simulink model "ARS308_RX"  (R2018b)
settings: Solver=FixedStepAuto  StartTime=0.0  StopTime=inf  FixedStep=0.005  RelTol=1e-3
PostLoadFcn:
  | if any(exist('dsrtsu_mdlpostloadfcn', 'file') ~= 0), dsrtsu_mdlpostloadfcn('Execute', bdroot); end
libraries: rtican x18
(part 1 of 4)
settings Model: DataDictionary=ARS308_RX.sldd  DSRTSU_INTERNAL_RTI_VER=540  DSRTSU_INTERNAL_RTI_TYPE=rti1401  RTICANMMDATA=struct('GeneralSetupData',struct('modelroot','F:\src_cm4sl_1221p\src_cm4sl_1221p\src_cm4sl','generalsettings',struct('filesettings',struct('destfolder',struct('Name','RTICANMM_FILES','Check',1),'buildfolder',struct('Name','.','Check',1),'AbsDestfolder',struct('Name','F:\src_cm4sl_1221p\src_cm4sl_1221p\src_cm4sl\RTICANMM_FILES'),'AbsBuildfolder',struct('Name','F:\src_cm4sl_1221p\src_cm4sl_1221p\src_cm4sl'))),'options',struct('addpaths',1,'rmpaths',1,'addtrcexclusion',logical(1),'cannavigator',struct('checkmonitoring',0),'show_usrtrc',0,'use_usrtrc',0),'advanced',struct('options',ones(1,100)),'MPSetup',{{}},'RTI',struct('Type','RTI1401','Ver','7.12','Date','02-May-2019'),'modelname','ARS308_RX','block','ARS308_RX'))  DSRTSU_INTERNAL_RTIFPGA=130  Creator=Administrator  LastModifiedBy=石丽
settings OptimizationCC: BlockReduction=off  ConditionallyExecuteInputs=off  OptimizeBlockIOStorage=off  BufferReuse=off  GlobalBufferReuse=off  ExpressionFolding=off  PassReuseOutputArgsThreshold=0  LocalBlockOutputs=off  OptimizeBlockOrder=speed  OptimizeDataStoreBuffers=off  BusAssignmentInplaceUpdate=off
settings DebuggingCC: ParameterTunabilityLossMsg=error  BusObjectLabelMismatch=none
settings HardwareCC: ProdBitPerPointer=32  ProdBitPerSizeT=32  ProdBitPerPtrDiffT=32  ProdLargestAtomicInteger=Integer  ProdEndianess=BigEndian  ProdWordSize=32  ProdHWDeviceType=Custom Processor->Custom  TargetIntDivRoundTo=Zero  TargetEndianess=BigEndian  TargetHWDeviceType=Custom Processor->Custom
settings ModelReferenceCC: ModelReferenceNumInstancesAllowed=Single
settings SFSimCC: MATLABDynamicMemAlloc=off
settings RTWCC: SystemTargetFile=rti1401.tlc  MakeCommand=make_rti  TemplateMakefile=rti1401.tmf  Description=dSPACE DS1401 Hardware Platform  GenerateReport=on  LaunchReport=on
settings CodeAppCC: OperatorAnnotations=on
settings STFCustomTargetCC: ParMdlRefBuildCompliant=on  SystemTargetFile=rti1401.tlc
settings GRTTargetCC: TargetLangStandard=C89/C90 (ANSI)  CompOptLevelCompliant=off  ConcurrentExecutionCompliant=off  CombineOutputUpdateFcns=off  MatFileLogging=off  CPPClassGenCompliant=off  UseToolchainInfoCompliant=off

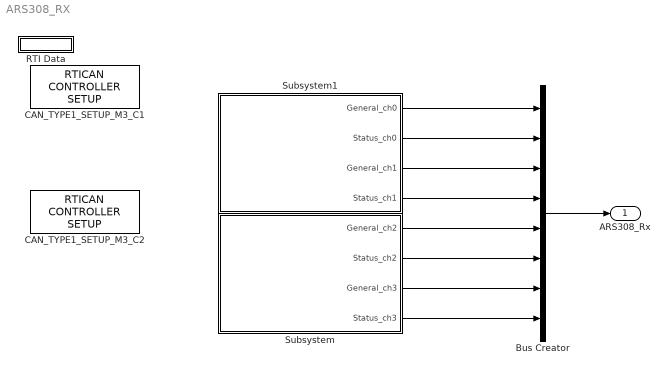
== system ARS308_RX ==
  Bus Creator : BusCreator  Inputs=8  OutDataTypeStr=Bus: ARS308_RX  NonVirtualBus=on
      settings: InheritFromInputs=off
  CAN_TYPE1_SETUP_M3_C1 : rtican/RTICAN CONTROLLER SETUP   Reserved1=[]  Reserved2=[]  Reserved3=[]  Reserved4=[]  AcceptanceMask=[]  ArbitrationField=[]  Parameters=[]  SFcnRTICANSettings=[]  MS_Struct=[]  BoardTypeNo=[]  BoardNo=[]  ChannelNo=[]  DialogFcn=[]  UnitName=[]  Revision=[]  UnitValues=[]  DSProperties=struct('RTI',struct('Version',uint32(12),'BlockType',struct('isSLSource',uint8(0),'isSLSink',uint8(0),'isHWSource',uint8(0),'isHWSink',uint8(0),'isSetup',uint8(1),'isInline',uint8(1),'isNonInline',uint8(0),'isInterrupt',uint8(0),'isChannelwise',uint8(0)),'IOBoardType','RTICAN','UnitType','NON_MESSAGE','Identifier','MASTER','DialogType','ML','BlockSet','RTICAN','SlaveProcessor','CAN'))  RTIBlockInterface=struct('InputPortsWidth',int32(0),'InputPortsActive',0,'OutputPortsWidth',int32(0),'OutputPortsActive',0,'DialogFcn','rtican_master_setup_gui','BlockDisplay',{{['CAN CONTROLLER\n SETUP'],'center'}},'IconTransparency','on','InitLevel',3,'IWork',{{{'',uint32(2)}}},'BlockName',struct('Token',{{'CAN_TYPE','_SETUP_M','_C'}},'BlockParam',{{'BoardTypeNo','BoardNo','ChannelNo'}}),'ParameterTunableNames',{{}})  RTIBlockParameters="struct('BoardTypeNo',{{1,'OFF',[]}},'BoardNo',{{3,'ON',[1 16]}},'ChannelNo',{{1,'ON',[1 2]}},'AcceptanceMask',{{0,'OFF',[]}},'ArbitrationField',{{0,'OFF',[]}},'Parameters',{{struct('Config',struct('Baudrate',500,'SampleMode',1,'UsedParamSet',1,'validSettings',1,'isBTRvalues',0,'Advanced',struct('Baudrate',{500,500,500},'Frequency',{24000000,36000000,64000000},'Settings',{struct('SMPL',0,'BRP',0,'NBT',24,'TSEG1',15,'TSEG2',6,'SJW',3,'SP',70),struct('SMPL',0,'BRP',1,'NBT',18,'TSEG1',14,'TSEG2',1,'SJW',1,'SP',88),struct('SMPL',0,'BRP',3,'NBT',16,'TSEG1',12,'TSEG2',1,'SJW',1,'SP',87)},'BTR0',{192,65,67},'BTR1',{111,30,28})),'configType',1,'Options',struct('DataFileSelected',1,'DataFileName',{{['c:\\users\\石丽\\desktop\\zone\\2020_demo\\308\\ars408_can_database_ch0 -new.dbc'],'c:\\users\\石丽\\desktop\\zone\\2020_demo\\308\\ars408_can_database_ch1-new.dbc'}},'DataFileDate',{{['18-12月-2020 14:05:27'],['18-12月-2020 14:05:27']}},'InterfaceFcn','rtican_dbc_file_parser','InterfaceFcnFileName','','LabelConfigType','volatile','AcceptanceMaskSelected',0,'MsgDataType','AllwaysDouble','NumType','hex','MaskType','STD','AcceptanceMask',0,'ArbitrationField',0,'UseMultipleMessageAccess',1),'RxReceiveStdOptions',struct('RxServiceStdEnabled',0,'RxServiceStdMsgIdent',1000,'RxServiceStdIdentNumType',1,'RxServiceStdIdentMask',0,'RxServiceStdMaskNumType',1,'RxServiceStdQueueSize',64),'RxReceiveXtdOptions',struct('RxServiceXtdEnabled',0,'RxServiceXtdMsgIdent',1001,'RxServiceXtdIdentNumType',1,'RxServiceXtdIdentMask',0,'RxServiceXtdMaskNumType',1,'RxServiceXtdQueueSize',64),'PartialNetworkingOptions',struct('switchedon',0,'format',1,'idmask',['    XXXXX XXXXXXXX XXXXXXXX XXXXXXXX'],'idcode','0','idfilter','0','datamaskused',0,'datalength',1,'datamask','0x0000000000000000','partialnetworkenable',0),'general',struct('Termination_common',1,'Termination_C252',1,'BusConfigurationRegister',0,'Transceiver','ISO11898','isFromLib',0)),'OFF',[]}},'CCPParameters',{{struct('CRO',struct('Format','STD','NumFormat','hex','Id',1639),'DTO',struct('Format','STD','NumFormat','hex','Id',2017),'StationAdr',struct('NumFormat','hex','Value',57),'StationId',struct('Value',['dSPACE CCP Service']),'Enabled',0),'OFF',[]}},'XCPParameters',{{struct('MASTER',struct('Format','STD','NumFormat','hex','Id',256),'SLAVE',struct('Format','STD','NumFormat','hex','Id',510),'Enabled',0,'PIDTransmissionEnabled',0),'OFF',[]}},'GroupId',{{struct('Group',{{'RTICAN'}},'No',2,'Behavior',{{'EVER'}},'BlockType',{{'SOURCE'}},'NameChangeFlag',1),'OFF',[]}},'SFcnRTICANSettings',{{struct('Baudrate',500,'configType',1,'AdvancedConfig',struct('Frequency',{},'BTR0',{},'BTR1',{}),'UsedParamSet',1,'STDMaskSelected','no','XTDMaskSelected','no','BoardType','DS1','BoardNo',3,'ControllerNo',1,'Transceiver','ISO11898','BusConfigRegister',0,'TerminationRes',120,'UseMultipleMessageAccess','yes','STDRXSrvcUsed','no','STDRXSrvcMsgId',1000,'STDRXSrvcMsgMask',0,'STDRXSrvcQueueSize',64,'XTDRXSrvcUsed','no','XTDRXSrvcMsgId',1001,'XTDRXSrvcQueueSize',64,'XTDRXSrvcMsgMask',0,'PN_IsPNTransciever',0,'PN_IsPNEnabled',0,'PN_MsgFormat',1,'PN_idcode',0,'PN_idmask',2047,'PN_datamaskused',0,'PN_datalength',0,'PN_datamask',['0xFF, 0xFF, 0xFF, 0xFF, 0xFF, 0xFF, 0xFF, 0xFF']),'OFF',[]}},'SFcnRTICCPSettings',{{struct('CRO',struct('Format','STD','NumFormat','hex','Id',1639),'DTO',struct('Format','STD','NumFormat','hex','Id',2017),'StationAdr',struct('NumFormat','hex','Value',57),'StationId',struct('Value',['dSPACE CCP Service']),'Enabled',0),'OFF',[]}},'SFcnRTIXCPSettings',{{struct('MASTER',struct('Format','STD','NumFormat','hex','Id',256),'SLAVE',struct('Format','STD','NumFormat','hex','Id',510),'Enabled',0,'PIDTransmissionEnabled',0),'OFF',[]}},'TLCFileName',{{'rtican_master_setup','OFF',[]}})"  RTISFcnParameters=struct('SFcnRTICANSettings','struct','SFcnRTICCPSettings','struct','SFcnRTIXCPSettings','struct','AcceptanceMask','int32','ArbitrationField','int32','TLCFileName','char')  RTIBlockParaDefault="struct('BoardTypeNo',4302,'BoardNo',1,'ChannelNo',1,'AcceptanceMask',0,'ArbitrationField',0,'Parameters',struct('Config',struct('Baudrate',500,'SampleMode',1,'UsedParamSet',1,'validSettings',1,'isBTRvalues',0,'Advanced',struct('Frequency',16000000,'BTR0',64,'BTR1',28,'Settings',struct('SMPL',0,'BRP',0,'NBT',16,'TSEG1',12,'TSEG2',1,'SJW',1,'SP',87))),'configType',1,'Options',struct('DataFileSelected',0,'DataFileName',{{['<no datafile support>']}},'DataFileDate',{{''}},'InterfaceFcn','rtican_dbc_file_parser','InterfaceFcnFileName','','LabelConfigType','volatile','AcceptanceMaskSelected',0,'MsgDataType','AllwaysDouble','NumType','hex','MaskType','STD','AcceptanceMask',0,'ArbitrationField',0,'UseMultipleMessageAccess',0),'RxReceiveStdOptions',struct('RxServiceStdEnabled',0,'RxServiceStdMsgIdent',1000,'RxServiceStdIdentNumType',1,'RxServiceStdIdentMask',0,'RxServiceStdMaskNumType',1,'RxServiceStdQueueSize',64),'RxReceiveXtdOptions',struct('RxServiceXtdEnabled',0,'RxServiceXtdMsgIdent',1001,'RxServiceXtdIdentNumType',1,'RxServiceXtdIdentMask',0,'RxServiceXtdMaskNumType',1,'RxServiceXtdQueueSize',64),'PartialNetworkingOptions',struct('switchedon',0,'format',1,'idmask',['    XXXXX XXXXXXXX XXXXXXXX XXXXXXXX'],'idcode','0','idfilter','0','datamaskused',0,'datalength',1,'datamask','0x0000000000000000','partialnetworkenable',0),'general',struct('Termination_common',1,'Termination_C252',1,'BusConfigurationRegister',0,'Transceiver','ISO11898','isFromLib',1)),'CCPParameters',struct('CRO',struct('Format','STD','NumFormat','hex','Id',1639),'DTO',struct('Format','STD','NumFormat','hex','Id',2017),'StationAdr',struct('NumFormat','hex','Value',57),'StationId',struct('Value',['dSPACE CCP Service']),'Enabled',0),'XCPParameters',struct('MASTER',struct('Format','STD','NumFormat','hex','Id',256),'SLAVE',struct('Format','STD','NumFormat','hex','Id',510),'Enabled',0,'PIDTransmissionEnabled',0),'GroupId',struct('Group',{{'RTICAN'}},'No',1,'Behavior',{{'EVER'}},'BlockType',{{'SOURCE'}},'NameChangeFlag',1),'SFcnRTICANSettings',struct('Baudrate',500,'configType',1,'AdvandedConfig',struct('Frequency',16000000,'BTR0','0x40','BTR1','0x1C'),'UsedParamSet',1,'STDMaskSelected','no','XTDMaskSelected','no','BoardType','DS4302','BoardNo',1,'ControllerNo',1,'Transceiver','ISO11898','BusConfigRegister',0,'TerminationRes',120,'UseMultipleMessageAccess','no','STDRXSrvcUsed','no','STDRXSrvcMsgId',1000,'STDRXSrvcMsgMask',0,'STDRXSrvcQueueSize',64,'XTDRXSrvcUsed','no','XTDRXSrvcMsgId',1001,'XTDRXSrvcQueueSize',64,'XTDRXSrvcMsgMask',0),'SFcnRTICCPSettings',struct('CRO',struct('Format','STD','NumFormat','hex','Id',1639),'DTO',struct('Format','STD','NumFormat','hex','Id',2017),'StationAdr',struct('NumFormat','hex','Value',57),'StationId',struct('Value',['dSPACE CCP Service']),'Enabled',0),'SFcnRTIXCPSettings',struct('MASTER',struct('Format','STD','NumFormat','hex','Id',256),'SLAVE',struct('Format','STD','NumFormat','hex','Id',510),'Enabled',0,'PIDTransmissionEnabled',0),'TLCFileName','rtican_master_setup')"
      settings: AttributesFormatString=Group Id: RTICAN2\n  SourceProductName=dSPACE RTI CAN Blockset
  CAN_TYPE1_SETUP_M3_C2 : rtican/RTICAN CONTROLLER SETUP   Reserved1=[]  Reserved2=[]  Reserved3=[]  Reserved4=[]  AcceptanceMask=[]  ArbitrationField=[]  Parameters=[]  SFcnRTICANSettings=[]  MS_Struct=[]  BoardTypeNo=[]  BoardNo=[]  ChannelNo=[]  DialogFcn=[]  UnitName=[]  Revision=[]  UnitValues=[]  DSProperties=struct('RTI',struct('Version',uint32(12),'BlockType',struct('isSLSource',uint8(0),'isSLSink',uint8(0),'isHWSource',uint8(0),'isHWSink',uint8(0),'isSetup',uint8(1),'isInline',uint8(1),'isNonInline',uint8(0),'isInterrupt',uint8(0),'isChannelwise',uint8(0)),'IOBoardType','RTICAN','UnitType','NON_MESSAGE','Identifier','MASTER','DialogType','ML','BlockSet','RTICAN','SlaveProcessor','CAN'))  RTIBlockInterface=struct('InputPortsWidth',int32(0),'InputPortsActive',0,'OutputPortsWidth',int32(0),'OutputPortsActive',0,'DialogFcn','rtican_master_setup_gui','BlockDisplay',{{['CAN CONTROLLER\n SETUP'],'center'}},'IconTransparency','on','InitLevel',3,'IWork',{{{'',uint32(2)}}},'BlockName',struct('Token',{{'CAN_TYPE','_SETUP_M','_C'}},'BlockParam',{{'BoardTypeNo','BoardNo','ChannelNo'}}),'ParameterTunableNames',{{}})  RTIBlockParameters="struct('BoardTypeNo',{{1,'OFF',[]}},'BoardNo',{{3,'ON',[1 16]}},'ChannelNo',{{2,'ON',[1 2]}},'AcceptanceMask',{{0,'OFF',[]}},'ArbitrationField',{{0,'OFF',[]}},'Parameters',{{struct('Config',struct('Baudrate',500,'SampleMode',1,'UsedParamSet',1,'validSettings',1,'isBTRvalues',0,'Advanced',struct('Baudrate',{500,500,500},'Frequency',{24000000,36000000,64000000},'Settings',{struct('SMPL',0,'BRP',0,'NBT',24,'TSEG1',15,'TSEG2',6,'SJW',3,'SP',70),struct('SMPL',0,'BRP',1,'NBT',18,'TSEG1',14,'TSEG2',1,'SJW',1,'SP',88),struct('SMPL',0,'BRP',3,'NBT',16,'TSEG1',12,'TSEG2',1,'SJW',1,'SP',87)},'BTR0',{192,65,67},'BTR1',{111,30,28})),'configType',1,'Options',struct('DataFileSelected',1,'DataFileName',{{['c:\\users\\石丽\\desktop\\zone\\2020_demo\\308\\ars408_can_database_ch2 -new.dbc'],'c:\\users\\石丽\\desktop\\zone\\2020_demo\\308\\ars408_can_database_ch3-new.dbc'}},'DataFileDate',{{['18-12月-2020 14:05:28'],['18-12月-2020 14:05:26']}},'InterfaceFcn','rtican_dbc_file_parser','InterfaceFcnFileName','','LabelConfigType','volatile','AcceptanceMaskSelected',0,'MsgDataType','AllwaysDouble','NumType','hex','MaskType','STD','AcceptanceMask',0,'ArbitrationField',0,'UseMultipleMessageAccess',1),'RxReceiveStdOptions',struct('RxServiceStdEnabled',0,'RxServiceStdMsgIdent',1000,'RxServiceStdIdentNumType',1,'RxServiceStdIdentMask',0,'RxServiceStdMaskNumType',1,'RxServiceStdQueueSize',64),'RxReceiveXtdOptions',struct('RxServiceXtdEnabled',0,'RxServiceXtdMsgIdent',1001,'RxServiceXtdIdentNumType',1,'RxServiceXtdIdentMask',0,'RxServiceXtdMaskNumType',1,'RxServiceXtdQueueSize',64),'PartialNetworkingOptions',struct('switchedon',0,'format',1,'idmask',['    XXXXX XXXXXXXX XXXXXXXX XXXXXXXX'],'idcode','0','idfilter','0','datamaskused',0,'datalength',1,'datamask','0x0000000000000000','partialnetworkenable',0),'general',struct('Termination_common',1,'Termination_C252',1,'BusConfigurationRegister',0,'Transceiver','ISO11898','isFromLib',0)),'OFF',[]}},'CCPParameters',{{struct('CRO',struct('Format','STD','NumFormat','hex','Id',1639),'DTO',struct('Format','STD','NumFormat','hex','Id',2017),'StationAdr',struct('NumFormat','hex','Value',57),'StationId',struct('Value',['dSPACE CCP Service']),'Enabled',0),'OFF',[]}},'XCPParameters',{{struct('MASTER',struct('Format','STD','NumFormat','hex','Id',256),'SLAVE',struct('Format','STD','NumFormat','hex','Id',510),'Enabled',0,'PIDTransmissionEnabled',0),'OFF',[]}},'GroupId',{{struct('Group',{{'RTICAN'}},'No',1,'Behavior',{{'EVER'}},'BlockType',{{'SOURCE'}},'NameChangeFlag',1),'OFF',[]}},'SFcnRTICANSettings',{{struct('Baudrate',500,'configType',1,'AdvancedConfig',struct('Frequency',{},'BTR0',{},'BTR1',{}),'UsedParamSet',1,'STDMaskSelected','no','XTDMaskSelected','no','BoardType','DS1','BoardNo',3,'ControllerNo',2,'Transceiver','ISO11898','BusConfigRegister',0,'TerminationRes',120,'UseMultipleMessageAccess','yes','STDRXSrvcUsed','no','STDRXSrvcMsgId',1000,'STDRXSrvcMsgMask',0,'STDRXSrvcQueueSize',64,'XTDRXSrvcUsed','no','XTDRXSrvcMsgId',1001,'XTDRXSrvcQueueSize',64,'XTDRXSrvcMsgMask',0,'PN_IsPNTransciever',0,'PN_IsPNEnabled',0,'PN_MsgFormat',1,'PN_idcode',0,'PN_idmask',2047,'PN_datamaskused',0,'PN_datalength',0,'PN_datamask',['0xFF, 0xFF, 0xFF, 0xFF, 0xFF, 0xFF, 0xFF, 0xFF']),'OFF',[]}},'SFcnRTICCPSettings',{{struct('CRO',struct('Format','STD','NumFormat','hex','Id',1639),'DTO',struct('Format','STD','NumFormat','hex','Id',2017),'StationAdr',struct('NumFormat','hex','Value',57),'StationId',struct('Value',['dSPACE CCP Service']),'Enabled',0),'OFF',[]}},'SFcnRTIXCPSettings',{{struct('MASTER',struct('Format','STD','NumFormat','hex','Id',256),'SLAVE',struct('Format','STD','NumFormat','hex','Id',510),'Enabled',0,'PIDTransmissionEnabled',0),'OFF',[]}},'TLCFileName',{{'rtican_master_setup','OFF',[]}})"  RTISFcnParameters=struct('SFcnRTICANSettings','struct','SFcnRTICCPSettings','struct','SFcnRTIXCPSettings','struct','AcceptanceMask','int32','ArbitrationField','int32','TLCFileName','char')  RTIBlockParaDefault="struct('BoardTypeNo',4302,'BoardNo',1,'ChannelNo',1,'AcceptanceMask',0,'ArbitrationField',0,'Parameters',struct('Config',struct('Baudrate',500,'SampleMode',1,'UsedParamSet',1,'validSettings',1,'isBTRvalues',0,'Advanced',struct('Frequency',16000000,'BTR0',64,'BTR1',28,'Settings',struct('SMPL',0,'BRP',0,'NBT',16,'TSEG1',12,'TSEG2',1,'SJW',1,'SP',87))),'configType',1,'Options',struct('DataFileSelected',0,'DataFileName',{{['<no datafile support>']}},'DataFileDate',{{''}},'InterfaceFcn','rtican_dbc_file_parser','InterfaceFcnFileName','','LabelConfigType','volatile','AcceptanceMaskSelected',0,'MsgDataType','AllwaysDouble','NumType','hex','MaskType','STD','AcceptanceMask',0,'ArbitrationField',0,'UseMultipleMessageAccess',0),'RxReceiveStdOptions',struct('RxServiceStdEnabled',0,'RxServiceStdMsgIdent',1000,'RxServiceStdIdentNumType',1,'RxServiceStdIdentMask',0,'RxServiceStdMaskNumType',1,'RxServiceStdQueueSize',64),'RxReceiveXtdOptions',struct('RxServiceXtdEnabled',0,'RxServiceXtdMsgIdent',1001,'RxServiceXtdIdentNumType',1,'RxServiceXtdIdentMask',0,'RxServiceXtdMaskNumType',1,'RxServiceXtdQueueSize',64),'PartialNetworkingOptions',struct('switchedon',0,'format',1,'idmask',['    XXXXX XXXXXXXX XXXXXXXX XXXXXXXX'],'idcode','0','idfilter','0','datamaskused',0,'datalength',1,'datamask','0x0000000000000000','partialnetworkenable',0),'general',struct('Termination_common',1,'Termination_C252',1,'BusConfigurationRegister',0,'Transceiver','ISO11898','isFromLib',1)),'CCPParameters',struct('CRO',struct('Format','STD','NumFormat','hex','Id',1639),'DTO',struct('Format','STD','NumFormat','hex','Id',2017),'StationAdr',struct('NumFormat','hex','Value',57),'StationId',struct('Value',['dSPACE CCP Service']),'Enabled',0),'XCPParameters',struct('MASTER',struct('Format','STD','NumFormat','hex','Id',256),'SLAVE',struct('Format','STD','NumFormat','hex','Id',510),'Enabled',0,'PIDTransmissionEnabled',0),'GroupId',struct('Group',{{'RTICAN'}},'No',1,'Behavior',{{'EVER'}},'BlockType',{{'SOURCE'}},'NameChangeFlag',1),'SFcnRTICANSettings',struct('Baudrate',500,'configType',1,'AdvandedConfig',struct('Frequency',16000000,'BTR0','0x40','BTR1','0x1C'),'UsedParamSet',1,'STDMaskSelected','no','XTDMaskSelected','no','BoardType','DS4302','BoardNo',1,'ControllerNo',1,'Transceiver','ISO11898','BusConfigRegister',0,'TerminationRes',120,'UseMultipleMessageAccess','no','STDRXSrvcUsed','no','STDRXSrvcMsgId',1000,'STDRXSrvcMsgMask',0,'STDRXSrvcQueueSize',64,'XTDRXSrvcUsed','no','XTDRXSrvcMsgId',1001,'XTDRXSrvcQueueSize',64,'XTDRXSrvcMsgMask',0),'SFcnRTICCPSettings',struct('CRO',struct('Format','STD','NumFormat','hex','Id',1639),'DTO',struct('Format','STD','NumFormat','hex','Id',2017),'StationAdr',struct('NumFormat','hex','Value',57),'StationId',struct('Value',['dSPACE CCP Service']),'Enabled',0),'SFcnRTIXCPSettings',struct('MASTER',struct('Format','STD','NumFormat','hex','Id',256),'SLAVE',struct('Format','STD','NumFormat','hex','Id',510),'Enabled',0,'PIDTransmissionEnabled',0),'TLCFileName','rtican_master_setup')"
      settings: AttributesFormatString=Group Id: RTICAN1\n  SourceProductName=dSPACE RTI CAN Blockset
  RTI Data : Subsystem  Tag=struct('RTIDataServer',struct('RTIDataServerVs','2','RTIModelDescription','struct(''main'',''ARS308_RX'',''sub'',''ARS308_RX'',''isMp'',0)'))  LoadFcn="if exist('rtidc'), try,  rtidc('DataHostBlockClbLoad', gcbh); catch, disp(['Warning: ''LoadFcn'' for RTI Data block failed: ' lasterr]); end, end,"  mask(RTI_DATA_HOST){}
      mask help:
      | RTI Data Block.
      | This block is used by RTI to store internal model-dependent data.
      | Please keep this block on the root level of the model. Deleting this block will result in data loss.
      |
      | NEVER DELETE OR COPY THIS BLOCK!
      settings: CopyFcn="if exist('rtidc'), try,  rtidc('DataHostBlockClbCopy', gcbh); catch, disp(['Warning: ''CopyFcn'' for RTI Data block failed: ' lasterr]); end, end,"  DeleteFcn="if exist('rtidc'), try,  rtidc('DataHostBlockClbDelete', gcbh); catch, disp(['Warning: ''DeleteFcn'' for RTI Data block failed: ' lasterr]); end, end,"  ModelCloseFcn="if exist('rtidc'), try,  rtidc('DataHostBlockClbModelClose', gcbh); catch, disp(['Warning: ''ModelCloseFcn'' for RTI Data block failed: ' lasterr]); end, end,"  PreSaveFcn="if exist('rtidc'), try,  rtidc('DataHostBlockClbPreSave', gcbh); catch, disp(['Warning: ''PreSaveFcn'' for RTI Data block failed: ' lasterr]); end, end,"  PostSaveFcn="if exist('rtidc'), try,  rtidc('DataHostBlockClbPostSave', gcbh); catch, disp(['Warning: ''PostSaveFcn'' for RTI Data block failed: ' lasterr]); end, end,"  NameChangeFcn="if exist('rtidc'), try,  rtidc('DataHostBlockClbNameChange', gcbh); catch, disp(['Warning: ''NameChangeFcn'' for RTI Data block failed: ' lasterr]); end, end,"
      mask Help:
      | RTI Data Block.
      | This block is used by RTI to store internal model-dependent data.
      | Please keep this block on the root level of the model. Deleting this block will result in data loss.
      | 
      | NEVER DELETE OR COPY THIS BLOCK!
      mask Display:
      | text(0.5, 0.5, 'RTI Data', 'HorizontalAlignment', 'center');
      | plot([1 0]);
  Subsystem : Subsystem
  Subsystem1 : Subsystem
  ARS308_Rx : Outport  OutDataTypeStr=Bus: ARS308_RX  BusOutputAsStruct=on
  wires:
  Subsystem/1(General_ch2) -> Bus Creator/5
  Subsystem/2(Status_ch2) -> Bus Creator/6
  Subsystem/3(General_ch3) -> Bus Creator/7
  Subsystem/4(Status_ch3) -> Bus Creator/8
  Subsystem1/4(Status_ch1) -> Bus Creator/4
  Subsystem1/3(General_ch1) -> Bus Creator/3
  Subsystem1/2(Status_ch0) -> Bus Creator/2
  Subsystem1/1(General_ch0) -> Bus Creator/1
  Bus Creator/1 -> ARS308_Rx/1

== system ARS308_RX/RTI Data ==
  RTI Data Store : Subsystem  Tag="struct('private',struct('version',struct('dsVer',uint32(2),'dsVerCreation',uint32(2),'RTI',struct('ver','7.12','type','RTI1401')),'access',struct('type','Model','isPerm',1,'created',['24-Dec-2020 09:28:53'],'modified',['28-Dec-2020 13:55:52'],'location','')),'public',struct('main',struct('data',[]),'sub',struct('name',{{'ARS308_RX'}},'data',{{struct('TH',struct('thTaskInfo',struct('taskType',{'TIMER','HWINT','TMRINT','SWINT','GLINT'},'tasksNumOf',{1,8,0,0,0},'srcIds',{{'TIMERA'},{'CAN1','CAN2','CAN3','CAN4','CAN6','CAN5','CAN8','CAN7'},{},{},{}},'taskNames',{{['Timer Task 1']},{'CAN_TYPE1_INT_M2_C2','_CAN_TYPE1_INT_M2_C2','__CAN_TYPE1_INT_M2_C2','___CAN_TYPE1_INT_M2_C2','CAN_TYPE1_INT_M2_C1','_CAN_TYPE1_INT_M2_C1','__CAN_TYPE1_INT_M2_C1','___CAN_TYPE1_INT_M2_C1'},{},{},{}})),'th_tc',struct('dataType',{'TASK','TASK','TASK','TASK','TASK','TASK','TASK','TASK','TASK'},'taskGroupId',{'','','','','','','','',''},'taskGroupList',{{},{},{},{},{},{},{},{},{}},'taskSchedulingPolicy',{'FCFS','FCFS','FCFS','FCFS','FCFS','FCFS','FCFS','FCFS','FCFS'},'taskType',{'TIMER','HWINT','HWINT','HWINT','HWINT','HWINT','HWINT','HWINT','HWINT'},'blkh',{-1,'test_308_all/Subsystem/CAN_TYPE1_INT_M2_C2','test_308_all/Subsystem/_CAN_TYPE1_INT_M2_C2','test_308_all/Subsystem/__CAN_TYPE1_INT_M2_C2','test_308_all/Subsystem/___CAN_TYPE1_INT_M2_C2','test_308_all/Subsystem1/CAN_TYPE1_INT_M2_C1','test_308_all/Subsystem1/_CAN_TYPE1_INT_M2_C1','test_308_all/Subsystem1/__CAN_TYPE1_INT_M2_C1','test_308_all/Subsystem1/___CAN_TYPE1_INT_M2_C1'},'srcId',{'TIMERA','CAN1','CAN2','CAN3','CAN4','CAN6','CAN5','CAN8','CAN7'},'srcSgnName',{['Timer A interrupt'],['CAN_TYPE1_M2_C2 RX Interrupt'],['CAN_TYPE1_M2_C2 RX Interrupt'],['CAN_TYPE1_M2_C2 RX Interrupt'],['CAN_TYPE1_M2_C2 RX Interrupt'],['CAN_TYPE1_M2_C1 RX Interrupt'],['CAN_TYPE1_M2_C1 RX Interrupt'],['CAN_TYPE1_M2_C1 RX Interrupt'],['CAN_TYPE1_M2_C1 RX Interrupt']},'srcCpuName',{'','','','','','','','',''},'taskName',{['Timer Task 1  [0.005] s'],'CAN_TYPE1_INT_M2_C2','_CAN_TYPE1_INT_M2_C2','__CAN_TYPE1_INT_M2_C2','___CAN_TYPE1_INT_M2_C2','CAN_TYPE1_INT_M2_C1','_CAN_TYPE1_INT_M2_C1','__CAN_TYPE1_INT_M2_C1','___CAN_TYPE1_INT_M2_C1'},'taskNameDisplayExt',{'','','','','','','','',''},'smplTime',{0.005,0,0,0,0,0,0,0,0},'smplTimeOffs',{0,0,0,0,0,0,0,0,0},'hasFixedPriority',{0,0,0,0,0,0,0,0,0},'priority',{9,6,5,8,7,1,2,3,4},'hasFixedOvc',{0,0,0,0,0,0,0,0,0},'ovcType',{1,1,1,1,1,1,1,1,1},'ovcMax',{1,1,1,1,1,1,1,1,1}),'tc_th',struct('dataType',{'TASK','TASK','TASK','TASK','TASK','TASK','TASK','TASK','TASK'},'taskGroupId',{'','','','','','','','',''},'taskGroupList',{{},{},{},{},{},{},{},{},{}},'taskSchedulingPolicy',{'FCFS','FCFS','FCFS','FCFS','FCFS','FCFS','FCFS','FCFS','FCFS'},'taskType',{'TIMER','HWINT','HWINT','HWINT','HWINT','HWINT','HWINT','HWINT','HWINT'},'blkh',{-1,'test_308_all/Subsystem/CAN_TYPE1_INT_M2_C2','test_308_all/Subsystem/_CAN_TYPE1_INT_M2_C2','test_308_all/Subsystem/__CAN_TYPE1_INT_M2_C2','test_308_all/Subsystem/___CAN_TYPE1_INT_M2_C2','test_308_all/Subsystem1/CAN_TYPE1_INT_M2_C1','test_308_all/Subsystem1/_CAN_TYPE1_INT_M2_C1','test_308_all/Subsystem1/__CAN_TYPE1_INT_M2_C1','test_308_all/Subsystem1/___CAN_TYPE1_INT_M2_C1'},'srcId',{'TIMERA','CAN1','CAN2','CAN3','CAN4','CAN6','CAN5','CAN8','CAN7'},'srcSgnName',{['Timer A interrupt'],['CAN_TYPE1_M2_C2 RX Interrupt'],['CAN_TYPE1_M2_C2 RX Interrupt'],['CAN_TYPE1_M2_C2 RX Interrupt'],['CAN_TYPE1_M2_C2 RX Interrupt'],['CAN_TYPE1_M2_C1 RX Interrupt'],['CAN_TYPE1_M2_C1 RX Interrupt'],['CAN_TYPE1_M2_C1 RX Interrupt'],['CAN_TYPE1_M2_C1 RX Interrupt']},'srcCpuName',{'','','','','','','','',''},'taskName',{['Timer Task 1  [0.005] s'],'CAN_TYPE1_INT_M2_C2','_CAN_TYPE1_INT_M2_C2','__CAN_TYPE1_INT_M2_C2','___CAN_TYPE1_INT_M2_C2','CAN_TYPE1_INT_M2_C1','_CAN_TYPE1_INT_M2_C1','__CAN_TYPE1_INT_M2_C1','___CAN_TYPE1_INT_M2_C1'},'taskNameDisplayExt',{'','','','','','','','',''},'smplTime',{0.005,0,0,0,0,0,0,0,0},'smplTimeOffs',{0,0,0,0,0,0,0,0,0},'hasFixedPriority',{0,0,0,0,0,0,0,0,0},'priority',{9,6,5,8,7,1,2,3,4},'hasFixedOvc',{0,0,0,0,0,0,0,0,0},'ovcType',{1,1,1,1,1,1,1,1,1},'ovcMax',{1,1,1,1,1,1,1,1,1}))}})))"  mask(RTI_DATA_STORE){}
      mask help:
      | RTI Data Store Block. This block is used by RTI to store internal model dependent data. Deleting this block will result in data loss.
      |
      | NEVER DELETE, COPY, OR MODIFY THIS BLOCK!
      mask Help:
      | RTI Data Store Block. This block is used by RTI to store internal model dependent data. Deleting this block will result in data loss.
      | 
      | NEVER DELETE, COPY, OR MODIFY THIS BLOCK!
      mask Display: text(0.5, 0.5, ' ', 'HorizontalAlignment', 'center');

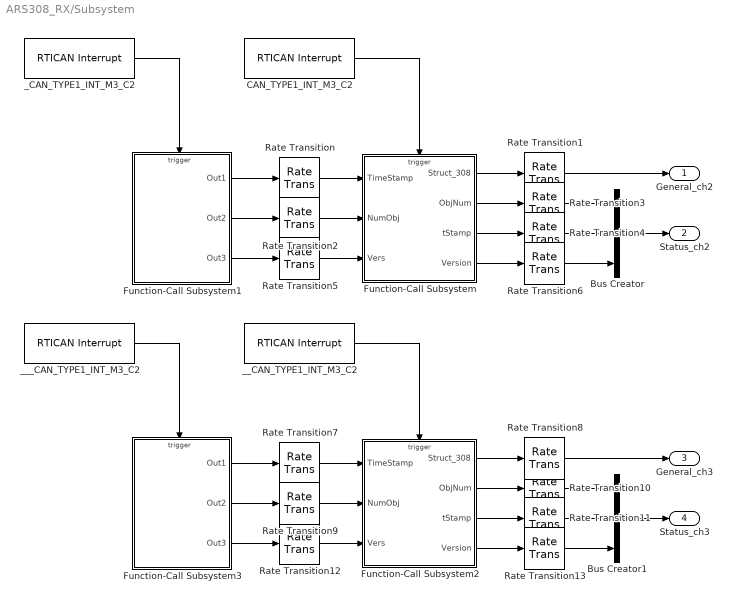
== system ARS308_RX/Subsystem ==
  Bus Creator : BusCreator  Inputs=3  OutDataTypeStr=Bus: Header_308  NonVirtualBus=on
      settings: InheritFromInputs=off
  Bus Creator1 : BusCreator  Inputs=3  OutDataTypeStr=Bus: Header_308  NonVirtualBus=on
      settings: InheritFromInputs=off
  CAN_TYPE1_INT_M3_C2 : rtican/RTICAN Interrupt  Reserved1=[]  Reserved2=[]  Reserved3=[]  Reserved4=[]  BoardTypeNo=[]  BoardNo=[]  ChannelNo=[]  Parameters=[]  InterruptName=[]  BoardIntNo=[]  Sfcn_Int_Struct=[]  BoardType=[]  SintNo=[]  Int_Struct=[]  DialogFcn=[]  UnitName=[]  Revision=[]  UnitValues=[]  DSProperties=struct('RTI',struct('Version',uint32(4),'BlockType',struct('isSLSource',uint8(1),'isSLSink',uint8(0),'isHWSource',uint8(1),'isHWSink',uint8(0),'isSetup',uint8(0),'isInline',uint8(1),'isNonInline',uint8(0),'isInterrupt',uint8(1),'isChannelwise',uint8(0)),'IOBoardType','RTICAN','UnitType','HWINT','Identifier','CANINT','DialogType','ML','BlockSet','RTICAN','RelationId',struct('TH',struct('BlockId','HWINT')),'SlaveProcessor','CAN'))  RTIBlockInterface=struct('OutputPortsWidth',int32(1),'FunctionCall',uint32(0),'OutputPortsActive',1,'DialogFcn','rtican_interrupt_gui','BlockDisplay',{{['CAN RX Interrupt'],'center'}},'IconTransparency','off','ParameterTunableNames',{{}},'InitLevel',3,'BlockName',struct('Token',{{'CAN_TYPE','_INT_M','_C'}},'BlockParam',{{'BoardTypeNo','BoardNo','ChannelNo'}}),'Options',{{'SS_OPTION_FORCE_NONINLINED_FCNCALL','SS_OPTION_ASYNCHRONOUS_INTERRUPT'}})  RTIBlockParameters=struct('BoardTypeNo',{{1,'OFF',[]}},'BoardNo',{{3,'ON',[1 16]}},'ChannelNo',{{2,'ON',[1 2]}},'Parameters',{{struct('general',struct('Type','RX','NumFormat','hex','MsgIdFormat','STD','MsgId',1579,'isFromLib',0)),'OFF',[]}},'GroupId',{{struct('Group','RTICAN','No',1,'Behavior','NAMECHANGE','BlockType','SINK','NameChangeFlag',0),'OFF',[]}},'SFcnRTICANInterrupt',{{0,'OFF',[]}},'ThSrcSgnName',{{['CAN_TYPE1_M3_C2 RX Interrupt'],'OFF',[]}},'ThBlk',{{['struct(''blkh'',''ARS308_RX/Subsystem/CAN_TYPE1_INT_M3_C2'',''srcId'',''CAN1'',''srcSgnId'',''CAN1'',''intervalTmrBlockId'',[],''srcSgnName'',[''CAN_TYPE1_M3_C2 RX Interrupt''],''srcCpuId'','''',''isSrcCpu'',1,''isTargetCpu'',1,''srcOnMasterCpu'',1,''boardType'',''CAN'',''boardTypeNo'',''1'',''boardNo'',2,''intNo'',0,''subIntNo'',-1,''period'',0,''entryPoint'',''rti_CAN1'',''blockName'',''CAN_TYPE1_INT_M3_C2'',''taskNameDisplayExt'','''',''taskType'',''HWINT'',''groupId'',''CANINT1B3'',''hookFcn'',''NULL'',''isTimerTaskSrc'',0,''service'','''',''mpBlkId'','''',''taskPriorityPreConfig'',''none'',''taskPriority'',-1,''taskSortWeighting'',[],''taskSchedulingPolicy'',''FCFS'',''taskOvrPreConfig'',''none'',''taskOvrStrategy'',1,''taskOvrQueueSize'',1,''taskVisibility'',''on'',''taskGroupId'','''',''taskGroupDisplayOrder'',[],''serviceDynamicGen'',0,''disableCodeGen'',0,''boardBase'',''0'',''noBoardBase'','''')'],'OFF',[]}},'PHSBoardBaseId',{{'DS4302','OFF',[]}},'TLCFileName',{{'rtican_interrupt','OFF',[]}})  RTISFcnParameters=struct('SFcnRTICANInterrupt','struct','ThBlk','struct','PHSBoardBaseId','char','TLCFileName','char')  RTIBlockParaDefault=struct('BoardTypeNo',4302,'BoardNo',1,'ChannelNo',1,'Parameters',struct('general',struct('Type','RX','NumFormat','dec','MsgIdFormat','STD','MsgId',100,'isFromLib',1)),'GroupId',struct('Group',{{'RTICAN'}},'No',1,'Behavior',{{'NAMECHANGE'}},'BlockType',{{'SINK'}},'NameChangeFlag',0),'SFcnRTICANInterrupt',0,'ThSrcSgnName',['DS4302CAN_B1_C1 RX Interrupt'],'ThBlk',['struct(''srcSgnId'', '''')'],'PHSBoardBaseId','DS4302','TLCFileName','rtican_interrupt')
      settings: AttributesFormatString=Group Id: RTICAN1\n  SourceProductName=dSPACE RTI CAN Blockset
  Function-Call Subsystem : Subsystem  TreatAsAtomicUnit=on
  Function-Call Subsystem1 : Subsystem  TreatAsAtomicUnit=on
  Function-Call Subsystem2 : Subsystem  TreatAsAtomicUnit=on
  Function-Call Subsystem3 : Subsystem  TreatAsAtomicUnit=on
  Rate Transition{,1..13} (14 alike) : RateTransition  Deterministic=off
  _CAN_TYPE1_INT_M3_C2 : rtican/RTICAN Interrupt  Reserved1=[]  Reserved2=[]  Reserved3=[]  Reserved4=[]  BoardTypeNo=[]  BoardNo=[]  ChannelNo=[]  Parameters=[]  InterruptName=[]  BoardIntNo=[]  Sfcn_Int_Struct=[]  BoardType=[]  SintNo=[]  Int_Struct=[]  DialogFcn=[]  UnitName=[]  Revision=[]  UnitValues=[]  DSProperties=struct('RTI',struct('Version',uint32(4),'BlockType',struct('isSLSource',uint8(1),'isSLSink',uint8(0),'isHWSource',uint8(1),'isHWSink',uint8(0),'isSetup',uint8(0),'isInline',uint8(1),'isNonInline',uint8(0),'isInterrupt',uint8(1),'isChannelwise',uint8(0)),'IOBoardType','RTICAN','UnitType','HWINT','Identifier','CANINT','DialogType','ML','BlockSet','RTICAN','RelationId',struct('TH',struct('BlockId','HWINT')),'SlaveProcessor','CAN'))  RTIBlockInterface=struct('OutputPortsWidth',int32(1),'FunctionCall',uint32(0),'OutputPortsActive',1,'DialogFcn','rtican_interrupt_gui','BlockDisplay',{{['CAN RX Interrupt'],'center'}},'IconTransparency','off','ParameterTunableNames',{{}},'InitLevel',3,'BlockName',struct('Token',{{'CAN_TYPE','_INT_M','_C'}},'BlockParam',{{'BoardTypeNo','BoardNo','ChannelNo'}}),'Options',{{'SS_OPTION_FORCE_NONINLINED_FCNCALL','SS_OPTION_ASYNCHRONOUS_INTERRUPT'}})  RTIBlockParameters=struct('BoardTypeNo',{{1,'OFF',[]}},'BoardNo',{{3,'ON',[1 16]}},'ChannelNo',{{2,'ON',[1 2]}},'Parameters',{{struct('general',struct('Type','RX','NumFormat','hex','MsgIdFormat','STD','MsgId',1578,'isFromLib',0)),'OFF',[]}},'GroupId',{{struct('Group','RTICAN','No',1,'Behavior','NAMECHANGE','BlockType','SINK','NameChangeFlag',0),'OFF',[]}},'SFcnRTICANInterrupt',{{0,'OFF',[]}},'ThSrcSgnName',{{['CAN_TYPE1_M3_C2 RX Interrupt'],'OFF',[]}},'ThBlk',{{['struct(''blkh'',''ARS308_RX/Subsystem/_CAN_TYPE1_INT_M3_C2'',''srcId'',''CAN2'',''srcSgnId'',''CAN2'',''intervalTmrBlockId'',[],''srcSgnName'',[''CAN_TYPE1_M3_C2 RX Interrupt''],''srcCpuId'','''',''isSrcCpu'',1,''isTargetCpu'',1,''srcOnMasterCpu'',1,''boardType'',''CAN'',''boardTypeNo'',''1'',''boardNo'',2,''intNo'',1,''subIntNo'',-1,''period'',0,''entryPoint'',''rti_CAN2'',''blockName'',''_CAN_TYPE1_INT_M3_C2'',''taskNameDisplayExt'','''',''taskType'',''HWINT'',''groupId'',''CANINT1B3'',''hookFcn'',''NULL'',''isTimerTaskSrc'',0,''service'','''',''mpBlkId'','''',''taskPriorityPreConfig'',''none'',''taskPriority'',-1,''taskSortWeighting'',[],''taskSchedulingPolicy'',''FCFS'',''taskOvrPreConfig'',''none'',''taskOvrStrategy'',1,''taskOvrQueueSize'',1,''taskVisibility'',''on'',''taskGroupId'','''',''taskGroupDisplayOrder'',[],''serviceDynamicGen'',0,''disableCodeGen'',0,''boardBase'',''0'',''noBoardBase'','''')'],'OFF',[]}},'PHSBoardBaseId',{{'DS4302','OFF',[]}},'TLCFileName',{{'rtican_interrupt','OFF',[]}})  RTISFcnParameters=struct('SFcnRTICANInterrupt','struct','ThBlk','struct','PHSBoardBaseId','char','TLCFileName','char')  RTIBlockParaDefault=struct('BoardTypeNo',4302,'BoardNo',1,'ChannelNo',1,'Parameters',struct('general',struct('Type','RX','NumFormat','dec','MsgIdFormat','STD','MsgId',100,'isFromLib',1)),'GroupId',struct('Group',{{'RTICAN'}},'No',1,'Behavior',{{'NAMECHANGE'}},'BlockType',{{'SINK'}},'NameChangeFlag',0),'SFcnRTICANInterrupt',0,'ThSrcSgnName',['DS4302CAN_B1_C1 RX Interrupt'],'ThBlk',['struct(''srcSgnId'', '''')'],'PHSBoardBaseId','DS4302','TLCFileName','rtican_interrupt')
      settings: AttributesFormatString=Group Id: RTICAN1\n  SourceProductName=dSPACE RTI CAN Blockset
  __CAN_TYPE1_INT_M3_C2 : rtican/RTICAN Interrupt  Reserved1=[]  Reserved2=[]  Reserved3=[]  Reserved4=[]  BoardTypeNo=[]  BoardNo=[]  ChannelNo=[]  Parameters=[]  InterruptName=[]  BoardIntNo=[]  Sfcn_Int_Struct=[]  BoardType=[]  SintNo=[]  Int_Struct=[]  DialogFcn=[]  UnitName=[]  Revision=[]  UnitValues=[]  DSProperties=struct('RTI',struct('Version',uint32(4),'BlockType',struct('isSLSource',uint8(1),'isSLSink',uint8(0),'isHWSource',uint8(1),'isHWSink',uint8(0),'isSetup',uint8(0),'isInline',uint8(1),'isNonInline',uint8(0),'isInterrupt',uint8(1),'isChannelwise',uint8(0)),'IOBoardType','RTICAN','UnitType','HWINT','Identifier','CANINT','DialogType','ML','BlockSet','RTICAN','RelationId',struct('TH',struct('BlockId','HWINT')),'SlaveProcessor','CAN'))  RTIBlockInterface=struct('OutputPortsWidth',int32(1),'FunctionCall',uint32(0),'OutputPortsActive',1,'DialogFcn','rtican_interrupt_gui','BlockDisplay',{{['CAN RX Interrupt'],'center'}},'IconTransparency','off','ParameterTunableNames',{{}},'InitLevel',3,'BlockName',struct('Token',{{'CAN_TYPE','_INT_M','_C'}},'BlockParam',{{'BoardTypeNo','BoardNo','ChannelNo'}}),'Options',{{'SS_OPTION_FORCE_NONINLINED_FCNCALL','SS_OPTION_ASYNCHRONOUS_INTERRUPT'}})  RTIBlockParameters=struct('BoardTypeNo',{{1,'OFF',[]}},'BoardNo',{{3,'ON',[1 16]}},'ChannelNo',{{2,'ON',[1 2]}},'Parameters',{{struct('general',struct('Type','RX','NumFormat','hex','MsgIdFormat','STD','MsgId',1595,'isFromLib',0)),'OFF',[]}},'GroupId',{{struct('Group','RTICAN','No',1,'Behavior','NAMECHANGE','BlockType','SINK','NameChangeFlag',0),'OFF',[]}},'SFcnRTICANInterrupt',{{0,'OFF',[]}},'ThSrcSgnName',{{['CAN_TYPE1_M3_C2 RX Interrupt'],'OFF',[]}},'ThBlk',{{['struct(''blkh'',''ARS308_RX/Subsystem/__CAN_TYPE1_INT_M3_C2'',''srcId'',''CAN3'',''srcSgnId'',''CAN3'',''intervalTmrBlockId'',[],''srcSgnName'',[''CAN_TYPE1_M3_C2 RX Interrupt''],''srcCpuId'','''',''isSrcCpu'',1,''isTargetCpu'',1,''srcOnMasterCpu'',1,''boardType'',''CAN'',''boardTypeNo'',''1'',''boardNo'',2,''intNo'',2,''subIntNo'',-1,''period'',0,''entryPoint'',''rti_CAN3'',''blockName'',''__CAN_TYPE1_INT_M3_C2'',''taskNameDisplayExt'','''',''taskType'',''HWINT'',''groupId'',''CANINT1B3'',''hookFcn'',''NULL'',''isTimerTaskSrc'',0,''service'','''',''mpBlkId'','''',''taskPriorityPreConfig'',''none'',''taskPriority'',-1,''taskSortWeighting'',[],''taskSchedulingPolicy'',''FCFS'',''taskOvrPreConfig'',''none'',''taskOvrStrategy'',1,''taskOvrQueueSize'',1,''taskVisibility'',''on'',''taskGroupId'','''',''taskGroupDisplayOrder'',[],''serviceDynamicGen'',0,''disableCodeGen'',0,''boardBase'',''0'',''noBoardBase'','''')'],'OFF',[]}},'PHSBoardBaseId',{{'DS4302','OFF',[]}},'TLCFileName',{{'rtican_interrupt','OFF',[]}})  RTISFcnParameters=struct('SFcnRTICANInterrupt','struct','ThBlk','struct','PHSBoardBaseId','char','TLCFileName','char')  RTIBlockParaDefault=struct('BoardTypeNo',4302,'BoardNo',1,'ChannelNo',1,'Parameters',struct('general',struct('Type','RX','NumFormat','dec','MsgIdFormat','STD','MsgId',100,'isFromLib',1)),'GroupId',struct('Group',{{'RTICAN'}},'No',1,'Behavior',{{'NAMECHANGE'}},'BlockType',{{'SINK'}},'NameChangeFlag',0),'SFcnRTICANInterrupt',0,'ThSrcSgnName',['DS4302CAN_B1_C1 RX Interrupt'],'ThBlk',['struct(''srcSgnId'', '''')'],'PHSBoardBaseId','DS4302','TLCFileName','rtican_interrupt')
      settings: AttributesFormatString=Group Id: RTICAN1\n  SourceProductName=dSPACE RTI CAN Blockset
  ___CAN_TYPE1_INT_M3_C2 : rtican/RTICAN Interrupt  Reserved1=[]  Reserved2=[]  Reserved3=[]  Reserved4=[]  BoardTypeNo=[]  BoardNo=[]  ChannelNo=[]  Parameters=[]  InterruptName=[]  BoardIntNo=[]  Sfcn_Int_Struct=[]  BoardType=[]  SintNo=[]  Int_Struct=[]  DialogFcn=[]  UnitName=[]  Revision=[]  UnitValues=[]  DSProperties=struct('RTI',struct('Version',uint32(4),'BlockType',struct('isSLSource',uint8(1),'isSLSink',uint8(0),'isHWSource',uint8(1),'isHWSink',uint8(0),'isSetup',uint8(0),'isInline',uint8(1),'isNonInline',uint8(0),'isInterrupt',uint8(1),'isChannelwise',uint8(0)),'IOBoardType','RTICAN','UnitType','HWINT','Identifier','CANINT','DialogType','ML','BlockSet','RTICAN','RelationId',struct('TH',struct('BlockId','HWINT')),'SlaveProcessor','CAN'))  RTIBlockInterface=struct('OutputPortsWidth',int32(1),'FunctionCall',uint32(0),'OutputPortsActive',1,'DialogFcn','rtican_interrupt_gui','BlockDisplay',{{['CAN RX Interrupt'],'center'}},'IconTransparency','off','ParameterTunableNames',{{}},'InitLevel',3,'BlockName',struct('Token',{{'CAN_TYPE','_INT_M','_C'}},'BlockParam',{{'BoardTypeNo','BoardNo','ChannelNo'}}),'Options',{{'SS_OPTION_FORCE_NONINLINED_FCNCALL','SS_OPTION_ASYNCHRONOUS_INTERRUPT'}})  RTIBlockParameters=struct('BoardTypeNo',{{1,'OFF',[]}},'BoardNo',{{3,'ON',[1 16]}},'ChannelNo',{{2,'ON',[1 2]}},'Parameters',{{struct('general',struct('Type','RX','NumFormat','hex','MsgIdFormat','STD','MsgId',1594,'isFromLib',0)),'OFF',[]}},'GroupId',{{struct('Group','RTICAN','No',1,'Behavior','NAMECHANGE','BlockType','SINK','NameChangeFlag',0),'OFF',[]}},'SFcnRTICANInterrupt',{{0,'OFF',[]}},'ThSrcSgnName',{{['CAN_TYPE1_M3_C2 RX Interrupt'],'OFF',[]}},'ThBlk',{{['struct(''blkh'',''ARS308_RX/Subsystem/___CAN_TYPE1_INT_M3_C2'',''srcId'',''CAN4'',''srcSgnId'',''CAN4'',''intervalTmrBlockId'',[],''srcSgnName'',[''CAN_TYPE1_M3_C2 RX Interrupt''],''srcCpuId'','''',''isSrcCpu'',1,''isTargetCpu'',1,''srcOnMasterCpu'',1,''boardType'',''CAN'',''boardTypeNo'',''1'',''boardNo'',2,''intNo'',3,''subIntNo'',-1,''period'',0,''entryPoint'',''rti_CAN4'',''blockName'',''___CAN_TYPE1_INT_M3_C2'',''taskNameDisplayExt'','''',''taskType'',''HWINT'',''groupId'',''CANINT1B3'',''hookFcn'',''NULL'',''isTimerTaskSrc'',0,''service'','''',''mpBlkId'','''',''taskPriorityPreConfig'',''none'',''taskPriority'',-1,''taskSortWeighting'',[],''taskSchedulingPolicy'',''FCFS'',''taskOvrPreConfig'',''none'',''taskOvrStrategy'',1,''taskOvrQueueSize'',1,''taskVisibility'',''on'',''taskGroupId'','''',''taskGroupDisplayOrder'',[],''serviceDynamicGen'',0,''disableCodeGen'',0,''boardBase'',''0'',''noBoardBase'','''')'],'OFF',[]}},'PHSBoardBaseId',{{'DS4302','OFF',[]}},'TLCFileName',{{'rtican_interrupt','OFF',[]}})  RTISFcnParameters=struct('SFcnRTICANInterrupt','struct','ThBlk','struct','PHSBoardBaseId','char','TLCFileName','char')  RTIBlockParaDefault=struct('BoardTypeNo',4302,'BoardNo',1,'ChannelNo',1,'Parameters',struct('general',struct('Type','RX','NumFormat','dec','MsgIdFormat','STD','MsgId',100,'isFromLib',1)),'GroupId',struct('Group',{{'RTICAN'}},'No',1,'Behavior',{{'NAMECHANGE'}},'BlockType',{{'SINK'}},'NameChangeFlag',0),'SFcnRTICANInterrupt',0,'ThSrcSgnName',['DS4302CAN_B1_C1 RX Interrupt'],'ThBlk',['struct(''srcSgnId'', '''')'],'PHSBoardBaseId','DS4302','TLCFileName','rtican_interrupt')
      settings: AttributesFormatString=Group Id: RTICAN1\n  SourceProductName=dSPACE RTI CAN Blockset
  General_ch2 : Outport  OutDataTypeStr=Bus: Bus_308
  Status_ch2 : Outport  Port=2  OutDataTypeStr=Bus: Header_308
  General_ch3 : Outport  Port=3  OutDataTypeStr=Bus: Bus_308
  Status_ch3 : Outport  Port=4  OutDataTypeStr=Bus: Header_308
  wires:
  Rate Transition9/1 -> Function-Call Subsystem2/2(NumObj)
  Rate Transition4/1 -> Bus Creator/2
  _CAN_TYPE1_INT_M3_C2/1 -> Function-Call Subsystem1/Trigger
  Bus Creator/1 -> Status_ch2/1
  Rate Transition3/1 -> Bus Creator/1
  Rate Transition13/1 -> Bus Creator1/3
  Rate Transition12/1 -> Function-Call Subsystem2/3(Vers)
  Function-Call Subsystem/4(Version) -> Rate Transition6/1
  ___CAN_TYPE1_INT_M3_C2/1 -> Function-Call Subsystem3/Trigger
  Function-Call Subsystem/2(ObjNum) -> Rate Transition3/1
  Rate Transition7/1 -> Function-Call Subsystem2/1(TimeStamp)
  __CAN_TYPE1_INT_M3_C2/1 -> Function-Call Subsystem2/Trigger
  Rate Transition/1 -> Function-Call Subsystem/1(TimeStamp)
  Function-Call Subsystem3/3(Out3) -> Rate Transition12/1
  Function-Call Subsystem2/3(tStamp) -> Rate Transition11/1
  Function-Call Subsystem3/2(Out2) -> Rate Transition9/1
  Rate Transition11/1 -> Bus Creator1/2
  Function-Call Subsystem3/1(Out1) -> Rate Transition7/1
  Function-Call Subsystem1/1(Out1) -> Rate Transition/1
  CAN_TYPE1_INT_M3_C2/1 -> Function-Call Subsystem/Trigger
  Function-Call Subsystem2/2(ObjNum) -> Rate Transition10/1
  Rate Transition2/1 -> Function-Call Subsystem/2(NumObj)
  Rate Transition10/1 -> Bus Creator1/1
  Bus Creator1/1 -> Status_ch3/1
  Rate Transition8/1 -> General_ch3/1
  Function-Call Subsystem/3(tStamp) -> Rate Transition4/1
  Function-Call Subsystem2/1(Struct_308) -> Rate Transition8/1
  Function-Call Subsystem2/4(Version) -> Rate Transition13/1
  Function-Call Subsystem1/2(Out2) -> Rate Transition2/1
  Rate Transition1/1 -> General_ch2/1
  Function-Call Subsystem/1(Struct_308) -> Rate Transition1/1
  Rate Transition5/1 -> Function-Call Subsystem/3(Vers)
  Rate Transition6/1 -> Bus Creator/3
  Function-Call Subsystem1/3(Out3) -> Rate Transition5/1
